simulink library "WaveformsLib"  (Simulink 7.7)
settings: Solver=ode45  SolverMode=SingleTasking  StartTime=0.0  StopTime=10.0  RelTol=1e-3
undefined symbols (not defined in the file or in its folder): etaZ, EX, gainZ, gammaZ, mgZ, tauFall, tauFZ, tauRise, tauRZ, tauX
libraries: SpikingLib x10, WaveformsLib x6, simulink x3
settings Model: Creator=jpalma  LastModifiedBy=jpalma

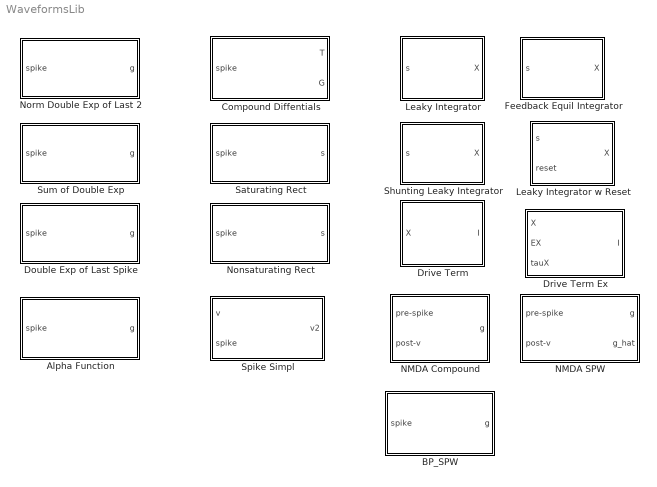
== system WaveformsLib ==
  Alpha Function : Subsystem  mask{tauDecay=2, onsetStr=1}
      mask prompts: tauDecay "Decay Time"; onsetStr "Onset Amplitude"
      mask help: Author: Jesse Palma
      mask Help: Author: Jesse Palma
      mask Display: image(imread('../Libs/icons/AlphaFunct.jpg'),'center');
  BP_SPW : Subsystem  mask{tRise=5, tFall=15, tBP=25, gBP=0.059}
      mask prompts: tRise "Tau Rise Time"; tFall "Tau Fall Time"; tBP "BP Width"; gBP "BP Gain"
      mask help:
      | dT/dt =  - T/tauRise + I * (1-T)
      | dG/dt =  - G/tauFall + T * (1-G)
      |
      | Author: Jesse Palma
      mask Help:
      | dT/dt =  - T/tauRise + I * (1-T)
      | dG/dt =  - G/tauFall + T * (1-G)
      | 
      | Author: Jesse Palma
      mask Display: image(imread('../Libs/icons/DoubleExp.jpg'),'center');
  Compound Diffentials : Subsystem  mask{tauRise=0.78, tauFall=6.5, squareWaveWidth=0.5, squareWaveHeight=2, interGain=1, finalGain=1}
      mask prompts: tauRise "Tau Rise Time"; tauFall "Tau Fall Time"; squareWaveWidth "Square Wave Width"; squareWaveHeight "Square Wave Height"; interGain "Intermediate Gain"; finalGain "Final Gain"
      mask help:
      | dT/dt =  - T/tauRise + I * (1-T)
      | dG/dt =  - G/tauFall + T * (1-G)
      |
      | Author: Jesse Palma
      mask Help:
      | dT/dt =  - T/tauRise + I * (1-T)
      | dG/dt =  - G/tauFall + T * (1-G)
      | 
      | Author: Jesse Palma
      mask Display: image(imread('../Libs/icons/DoubleExp.jpg'),'center');
  Double Exp of Last Spike : Subsystem  mask{tauRise=1, tauFall=2}
      mask prompts: tauRise "Tau Rise Time"; tauFall "Tau Fall Time"
      mask help: Author: Jesse Palma
      mask Help: Author: Jesse Palma
      mask Display: image(imread('../Libs/icons/DoubleExp.jpg'),'center');
  Drive Term : Subsystem  mask{EX=EX, tauX=tauX}
      mask prompts: EX "Equilibrium, EX"; tauX "Rate Time Constant, tauX"
      mask help: IX = 1/tauX (EX - X)
      mask Help: IX =  1/tauX (EX - X)
      mask Display: image(imread('../Libs/icons/DriveArrow.jpg'),'center');
  Drive Term Ex : Subsystem
      mask Description: IX =  1/tauX (EX - X)
      mask Help: IX =  1/tauX (EX - X)
      mask Display: image(imread('../Libs/icons/DriveArrow.jpg'),'center');
  Feedback Equil Integrator : Subsystem  mask{X0=0, A=0.05, EX=0}
      mask prompts: X0 "Initial Value, X0"; A "Decay Rate, A"; EX "Equilbrium (Rest) Value, EX"
      mask help:
      | dX/dt =  - A(EX - X) + s
      |
      | Author: Jesse Palma
      mask Help:
      | dX/dt =  - A(EX - X) + s
      | 
      | Author: Jesse Palma
      mask Display: image(imread('../Libs/icons/FeedbackEq.jpg'),'center');
  Leaky Integrator : Subsystem  mask{X0=0, A=0.05}
      mask prompts: X0 "Initial Value, X0"; A "Decay Rate, A"
      mask help: Author: Jesse Palma
      mask Help: Author: Jesse Palma
      mask Display: image(imread('../Libs/icons/Leaky.jpg'),'center');
  Leaky Integrator w Reset : Subsystem  mask{X0=0, A=0.05}
      mask prompts: X0 "Initial Value, X0"; A "Decay Rate, A"
      mask help: Author: Jesse Palma
      mask Help: Author: Jesse Palma
      mask Display: image(imread('../Libs/icons/Leaky.jpg'),'center');
  NMDA Compound : Subsystem  mask{rt=0.5, ft=40, eta=0.33, mg=1, gamma=0.06, gn=4}
      mask prompts: rt "Rise Time"; ft "Fall Time"; eta "Voltage-dependence, eta"; mg "Mg concentration"; gamma "Voltage-chandge-dependence, gamma"; gn "Concentration Gain, gN"
      mask Display: image(imread('../Libs/icons/DoubleExp.jpg'),'center');
  NMDA SPW : Subsystem  mask{tRise=tauRZ, tFall=tauFZ, eta=etaZ, mg=mgZ, gamma=gammaZ, gn=gainZ}
      mask prompts: tRise "Rise Time"; tFall "Fall Time"; eta "Voltage-dependence, eta"; mg "Mg concentration"; gamma "Voltage-chandge-dependence, gamma"; gn "Concentration Gain, gN"
      mask Display: image(imread('../Libs/icons/DoubleExp.jpg'),'center');
  Nonsaturating Rect : Subsystem  AncestorBlock=SpikeToWavesLib/Saturating Rectangular Wave  mask{squareWidth=1, squareHeight=1}
      mask prompts: squareWidth "Rectangular Width"; squareHeight "Rectangular Height"
      mask help: Author: Jesse Palma
      mask Help: Author: Jesse Palma
      mask Display: image(imread('../Libs/icons/SquareWave.jpg'),'center');
  Norm Double Exp of Last 2 : Subsystem  mask{tauRise=tauRise, tauFall=tauFall}
      mask prompts: tauRise "Tau Rise Time"; tauFall "Tau Fall Time"
      mask help:
      | Kinness Style
      |
      | Author: Jesse Palma
      mask Help:
      | Kinness Style
      | 
      | Author: Jesse Palma
      mask Display: image(imread('../Libs/icons/DoubleExp.jpg'),'center');
  Saturating Rect : Subsystem  mask{squareWidth=1, squareHeight=1}
      mask prompts: squareWidth "Rectangular Width"; squareHeight "Rectangular Height"
      mask help: Author: Jesse Palma
      mask Help: Author: Jesse Palma
      mask Display: image(imread('../Libs/icons/SquareWave.jpg'),'center');
  Shunting Leaky Integrator : Subsystem  mask{X0=0, A=0.05, B=1}
      mask prompts: X0 "Initial Value, X0"; A "Decay Rate, A"; B "Saturation Value, B"
      mask help: Author: Jesse Palma
      mask Help: Author: Jesse Palma
      mask Display: image(imread('../Libs/icons/SLeaky.jpg'),'center');
  Spike Simpl : Subsystem  mask{a=-0.2, b=0.65, c=0.002}
      mask prompts: a "A, drop slope"; b "B, max"; c "C, recovery slope"
      mask help: Author: Jesse Palma
      mask Help: Author: Jesse Palma
      mask Display: image(imread('../Libs/icons/SpikeSimp1.jpg'),'center');
  Sum of Double Exp : Subsystem  mask{tauRise=0.78, tauFall=6.5, timeStep=0.01}
      mask prompts: tauRise "Tau Rise Time"; tauFall "Tau Fall Time"; timeStep "Time Step"
      mask help: Author: Jesse Palma
      mask Help: Author: Jesse Palma
      mask Display: image(imread('../Libs/icons/DoubleExp.jpg'),'center');

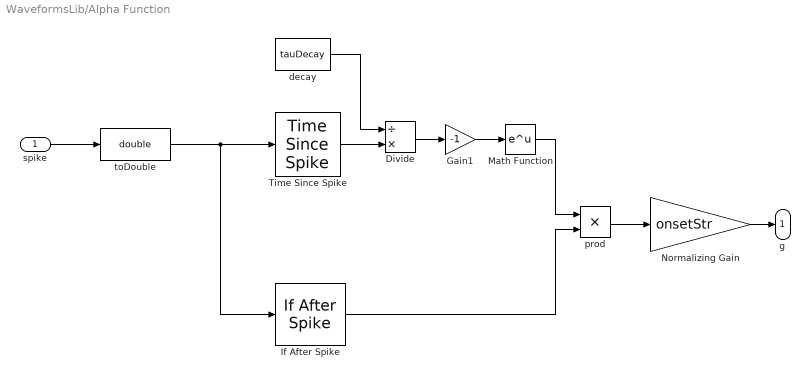
== system WaveformsLib/Alpha Function ==
  spike : Inport
  Divide : Product  Inputs=/*
  Gain1 : Gain  Gain=-1
  If After Spike : SpikingLib/If After Spike  SystemSampleTime=-1
  Math Function : Math  SaturateOnIntegerOverflow=on
  Normalizing Gain : Gain  Gain=onsetStr
  Time Since Spike : SpikingLib/Time Since Spike  SystemSampleTime=-1
  decay : Constant  Value=tauDecay
  prod : Product  Inputs=**
  toDouble : DataTypeConversion  OutDataTypeStr=double
  g : Outport
  wires:
  Normalizing Gain/1 -> g/1
  prod/1 -> Normalizing Gain/1
  spike/1 -> toDouble/1
  toDouble/1 -> Time Since Spike/1, If After Spike/1
  Gain1/1 -> Math Function/1
  Divide/1 -> Gain1/1
  decay/1 -> Divide/1
  Time Since Spike/1 -> Divide/2
  Math Function/1 -> prod/1
  If After Spike/1 -> prod/2

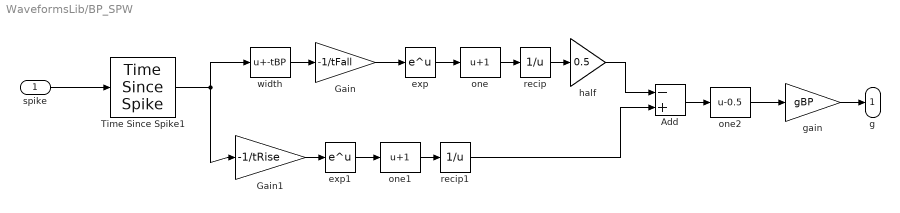
== system WaveformsLib/BP_SPW ==
  spike : Inport
  Add : Sum  Inputs=-+
  Gain : Gain  Gain=-1/tFall
  Gain1 : Gain  Gain=-1/tRise
  Time Since Spike1 : SpikingLib/Time Since Spike  SystemSampleTime=-1
  exp : Math  SaturateOnIntegerOverflow=on
  exp1 : Math  SaturateOnIntegerOverflow=on
  gain : Gain  Gain=gBP
  half : Gain  Gain=0.5
  one : Bias  Bias=1
  one1 : Bias  Bias=1
  one2 : Bias  Bias=-0.5
  recip : Math  Operator=reciprocal  SaturateOnIntegerOverflow=on
  recip1 : Math  Operator=reciprocal  SaturateOnIntegerOverflow=on
  width : Bias  Bias=-tBP
  g : Outport
  wires:
  spike/1 -> Time Since Spike1/1
  width/1 -> Gain/1
  Time Since Spike1/1 -> width/1, Gain1/1
  Gain/1 -> exp/1
  exp/1 -> one/1
  one/1 -> recip/1
  one1/1 -> recip1/1
  exp1/1 -> one1/1
  Gain1/1 -> exp1/1
  recip/1 -> half/1
  recip1/1 -> Add/2
  half/1 -> Add/1
  Add/1 -> one2/1
  one2/1 -> gain/1
  gain/1 -> g/1

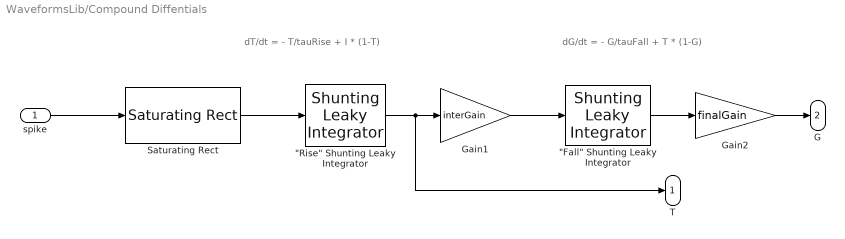
== system WaveformsLib/Compound Diffentials ==
  note: dT/dt = - T/tauRise + I * (1-T)
  note: dG/dt = - G/tauFall + T * (1-G)
  spike : Inport
  "\"Fall\" Shunting Leaky Integrator" : WaveformsLib/Shunting Leaky Integrator  SystemSampleTime=-1  X0=0  A=1/tauFall  B=1
  "\"Rise\" Shunting Leaky Integrator" : WaveformsLib/Shunting Leaky Integrator  SystemSampleTime=-1  X0=0  A=1/tauRise  B=1
  Gain1 : Gain  Gain=interGain
  Gain2 : Gain  Gain=finalGain
  Saturating Rect : WaveformsLib/Saturating Rect  SystemSampleTime=-1  squareWidth=squareWaveWidth  squareHeight=squareWaveHeight
  T : Outport
  G : Outport  Port=2
  wires:
  Gain2/1 -> G/1
  spike/1 -> Saturating Rect/1
  Saturating Rect/1 -> "\"Rise\" Shunting Leaky Integrator"/1
  "\"Rise\" Shunting Leaky Integrator"/1 -> Gain1/1, T/1
  Gain1/1 -> "\"Fall\" Shunting Leaky Integrator"/1
  "\"Fall\" Shunting Leaky Integrator"/1 -> Gain2/1

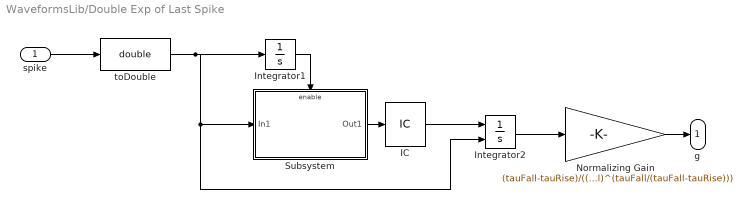
== system WaveformsLib/Double Exp of Last Spike ==
  spike : Inport
  IC : InitialCondition  Value=0
  Integrator1 : Integrator
  Integrator2 : Integrator  ExternalReset=rising
  Normalizing Gain : Gain  Gain=(tauFall-tauRise)/((tauRise/tauFall)^(tauRise/(tauFall-tauRise)) - (tauRise/tauFall)^(tauFall/(tauFall-tauRise)))
  Subsystem : Subsystem
  toDouble : DataTypeConversion  OutDataTypeStr=double
  g : Outport
  wires:
  Integrator1/1 -> Subsystem/Enable
  IC/1 -> Integrator2/1
  toDouble/1 -> Integrator2/2, Subsystem/1(In1), Integrator1/1
  spike/1 -> toDouble/1
  Subsystem/1(Out1) -> IC/1
  Integrator2/1 -> Normalizing Gain/1
  Normalizing Gain/1 -> g/1

== system WaveformsLib/Drive Term ==
  note: I_{X} = 1/tau_{X} (E_{X} - X)
  X : Inport
  XEq1 : Bias  Bias=-EX
  XGain : Gain  Gain=-1/tauX
  I : Outport
  wires:
  XGain/1 -> I/1
  XEq1/1 -> XGain/1
  X/1 -> XEq1/1

== system WaveformsLib/Drive Term Ex ==
  note: I_{X} = 1/tau_{X} (E_{X} - X)
  X : Inport
  EX : Inport  Port=2
  tauX : Inport  Port=3
  Add : Sum  Inputs=-+
  Product : Product  Inputs=*/  RndMeth=Zero
  I : Outport
  wires:
  X/1 -> Add/1
  EX/1 -> Add/2
  Product/1 -> I/1
  Add/1 -> Product/1
  tauX/1 -> Product/2

== system WaveformsLib/Feedback Equil Integrator ==
  note: dX/dt = - A(E_X - X) + s
  s : Inport
  Add : Sum  Inputs=+-
  Drive Term : WaveformsLib/Drive Term  SystemSampleTime=-1  EX=EX  tauX=1/A
  Integrate X : Integrator  InitialCondition=X0
  X : Outport
  wires:
  s/1 -> Add/1
  Integrate X/1 -> X/1, Drive Term/1
  Add/1 -> Integrate X/1
  Drive Term/1 -> Add/2

== system WaveformsLib/Leaky Integrator ==
  note: dX/dt = - AX + s
  note: Decay
  s : Inport
  Add : Sum  Inputs=+-
  Gain1 : Gain  Gain=A
  Integrate X : Integrator  InitialCondition=X0
  X : Outport
  wires:
  Gain1/1 -> Add/2
  Add/1 -> Integrate X/1
  Integrate X/1 -> Gain1/1, X/1
  s/1 -> Add/1

== system WaveformsLib/Leaky Integrator w Reset ==
  note: Decay
  note: dX/dt = - AX + s
  s : Inport
  reset : Inport  Port=2
  Add : Sum  Inputs=+-
  Gain1 : Gain  Gain=A
  Integrate X : Integrator  ExternalReset=falling  InitialCondition=X0
  X : Outport
  wires:
  s/1 -> Add/1
  Integrate X/1 -> X/1, Gain1/1
  Add/1 -> Integrate X/1
  Gain1/1 -> Add/2
  reset/1 -> Integrate X/2

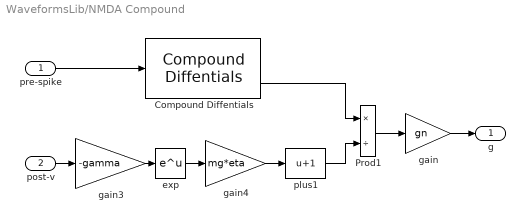
== system WaveformsLib/NMDA Compound ==
  pre-spike : Inport
  post-v : Inport  Port=2
  Compound Diffentials : WaveformsLib/Compound Diffentials  SystemSampleTime=-1  tauRise=rt  tauFall=ft  squareWaveWidth=0.5  squareWaveHeight=2  interGain=1  finalGain=1
  Prod1 : Product  Inputs=*/  RndMeth=Zero
  exp : Math  SaturateOnIntegerOverflow=on
  gain : Gain  Gain=gn
  gain3 : Gain  Gain=-gamma
  gain4 : Gain  Gain=mg*eta
  plus1 : Bias  Bias=1
  g : Outport
  wires:
  Compound Diffentials/2 -> Prod1/1
  gain3/1 -> exp/1
  exp/1 -> gain4/1
  gain4/1 -> plus1/1
  plus1/1 -> Prod1/2
  Prod1/1 -> gain/1
  pre-spike/1 -> Compound Diffentials/1
  post-v/1 -> gain3/1
  gain/1 -> g/1

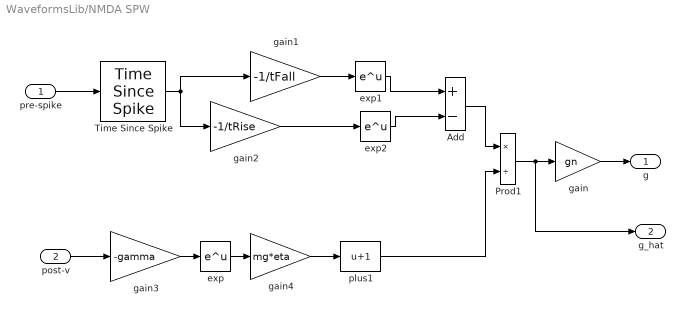
== system WaveformsLib/NMDA SPW ==
  pre-spike : Inport
  post-v : Inport  Port=2
  Add : Sum  Inputs=+-
  Prod1 : Product  Inputs=*/  RndMeth=Zero
  Time Since Spike : SpikingLib/Time Since Spike  SystemSampleTime=-1
  exp : Math  SaturateOnIntegerOverflow=on
  exp1 : Math  SaturateOnIntegerOverflow=on
  exp2 : Math  SaturateOnIntegerOverflow=on
  gain : Gain  Gain=gn
  gain1 : Gain  Gain=-1/tFall
  gain2 : Gain  Gain=-1/tRise
  gain3 : Gain  Gain=-gamma
  gain4 : Gain  Gain=mg*eta
  plus1 : Bias  Bias=1
  g : Outport
  g_hat : Outport  Port=2
  wires:
  gain/1 -> g/1
  post-v/1 -> gain3/1
  pre-spike/1 -> Time Since Spike/1
  Prod1/1 -> gain/1, g_hat/1
  plus1/1 -> Prod1/2
  gain4/1 -> plus1/1
  exp/1 -> gain4/1
  gain3/1 -> exp/1
  Add/1 -> Prod1/1
  gain1/1 -> exp1/1
  gain2/1 -> exp2/1
  exp1/1 -> Add/1
  exp2/1 -> Add/2
  Time Since Spike/1 -> gain1/1, gain2/1

== system WaveformsLib/Nonsaturating Rect ==
  spike : Inport
  Gain : Gain  Gain=squareHeight
  SpikeCounter : SpikingLib/SpikeCounter  SystemSampleTime=-1
  Subtract : Sum  Inputs=+-
  Transport Delay : TransportDelay  DelayTime=squareWidth
  s : Outport
  wires:
  Gain/1 -> s/1
  spike/1 -> SpikeCounter/1
  SpikeCounter/1 -> Subtract/1, Transport Delay/1
  Transport Delay/1 -> Subtract/2
  Subtract/1 -> Gain/1

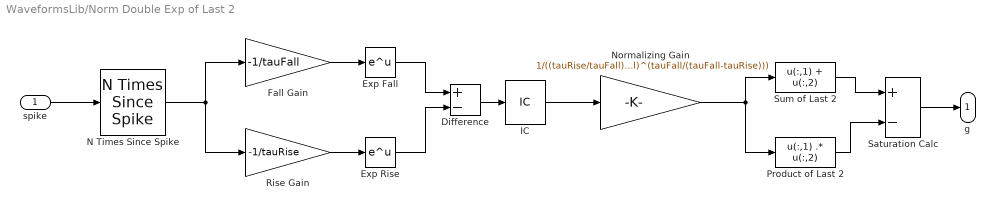
== system WaveformsLib/Norm Double Exp of Last 2 ==
  spike : Inport
  Difference : Sum  Inputs=+-
  Exp Fall : Math  SaturateOnIntegerOverflow=on
  Exp Rise : Math  SaturateOnIntegerOverflow=on
  Fall Gain : Gain  Gain=-1/tauFall
  IC : InitialCondition  Value=0
  N Times Since Spike : SpikingLib/N Times Since Spike  SystemSampleTime=-1  spikesMemory=2
  Normalizing Gain : Gain  Gain=1/((tauRise/tauFall)^(tauRise/(tauFall-tauRise)) - (tauRise/tauFall)^(tauFall/(tauFall-tauRise)))
  Product of Last 2 : MATLABFcn  MATLABFcn="u(:,1) .*  u(:,2)"
  Rise Gain : Gain  Gain=-1/tauRise
  Saturation Calc : Sum  Inputs=+-
  Sum of Last 2 : MATLABFcn  MATLABFcn=u(:,1) + u(:,2)
  g : Outport
  wires:
  Product of Last 2/1 -> Saturation Calc/2
  Sum of Last 2/1 -> Saturation Calc/1
  Normalizing Gain/1 -> Product of Last 2/1, Sum of Last 2/1
  Exp Rise/1 -> Difference/2
  Exp Fall/1 -> Difference/1
  Fall Gain/1 -> Exp Fall/1
  Rise Gain/1 -> Exp Rise/1
  Saturation Calc/1 -> g/1
  spike/1 -> N Times Since Spike/1
  IC/1 -> Normalizing Gain/1
  Difference/1 -> IC/1
  N Times Since Spike/1 -> Rise Gain/1, Fall Gain/1

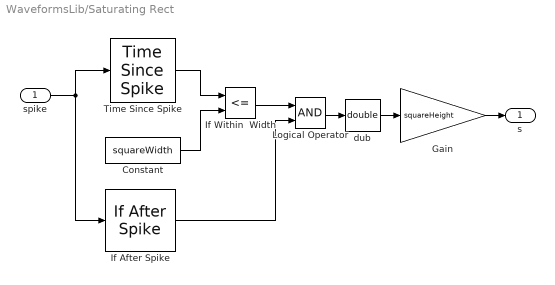
== system WaveformsLib/Saturating Rect ==
  spike : Inport
  Constant : Constant  Value=squareWidth
  Gain : Gain  Gain=squareHeight
  If After Spike : SpikingLib/If After Spike  SystemSampleTime=-1
  If Within  Width : RelationalOperator  Operator=<=  OutDataTypeStr=boolean
  Logical Operator : Logic  AllPortsSameDT=off  OutDataTypeStr=boolean
  Time Since Spike : SpikingLib/Time Since Spike  SystemSampleTime=-1
  dub : DataTypeConversion  OutDataTypeStr=double
  s : Outport
  wires:
  Logical Operator/1 -> dub/1
  Constant/1 -> If Within  Width/2
  If After Spike/1 -> Logical Operator/2
  If Within  Width/1 -> Logical Operator/1
  Time Since Spike/1 -> If Within  Width/1
  spike/1 -> Time Since Spike/1, If After Spike/1
  Gain/1 -> s/1
  dub/1 -> Gain/1

== system WaveformsLib/Shunting Leaky Integrator ==
  note: dX/dt = - AX + s * (B-X)
  s : Inport
  Leaky Integrator : WaveformsLib/Leaky Integrator  SystemSampleTime=-1  X0=X0  A=A
  Max Bias : Bias  Bias=B
  Product : Product  RndMeth=Zero
  Unary Minus : UnaryMinus
  X : Outport
  wires:
  s/1 -> Product/1
  Leaky Integrator/1 -> X/1, Unary Minus/1
  Product/1 -> Leaky Integrator/1
  Unary Minus/1 -> Max Bias/1
  Max Bias/1 -> Product/2

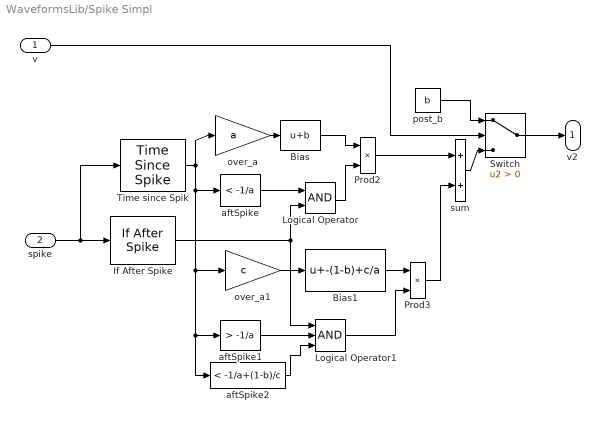
== system WaveformsLib/Spike Simpl ==
  v : Inport
  spike : Inport  Port=2
  Bias : Bias  Bias=b
  Bias1 : Bias  Bias=-(1-b)+c/a
  If After Spike : SpikingLib/If After Spike  SystemSampleTime=-1
  Logical Operator : Logic  AllPortsSameDT=off  OutDataTypeStr=boolean
  Logical Operator1 : Logic  Inputs=3  AllPortsSameDT=off  OutDataTypeStr=boolean
  Prod2 : Product  RndMeth=Zero
  Prod3 : Product  RndMeth=Zero
  Switch : Switch  Criteria=u2 > Threshold  ZeroCross=off
  Time since Spik : SpikingLib/Time Since Spike  SystemSampleTime=-1
  aftSpike : simulink/Logic and Bit Operations/Compare To Constant  SystemSampleTime=-1  relop=<  const=-1/a  LogicOutDataTypeMode=uint8  ZeroCross=off
  aftSpike1 : simulink/Logic and Bit Operations/Compare To Constant  SystemSampleTime=-1  relop=>  const=-1/a  LogicOutDataTypeMode=uint8  ZeroCross=off
  aftSpike2 : simulink/Logic and Bit Operations/Compare To Constant  SystemSampleTime=-1  relop=<  const=-1/a+(1-b)/c  LogicOutDataTypeMode=uint8  ZeroCross=off
  over_a : Gain  Gain=a
  over_a1 : Gain  Gain=c
  post_b : Constant  Value=b
  sum : Sum
  v2 : Outport
  wires:
  Switch/1 -> v2/1
  v/1 -> Switch/2
  Time since Spik/1 -> over_a/1, aftSpike/1, over_a1/1, aftSpike1/1, aftSpike2/1
  over_a/1 -> Bias/1
  Bias/1 -> Prod2/1
  aftSpike/1 -> Logical Operator/1
  If After Spike/1 -> Logical Operator/2, Logical Operator1/1
  Logical Operator/1 -> Prod2/2
  over_a1/1 -> Bias1/1
  aftSpike2/1 -> Logical Operator1/3
  aftSpike1/1 -> Logical Operator1/2
  Bias1/1 -> Prod3/1
  Logical Operator1/1 -> Prod3/2
  Prod3/1 -> sum/2
  Prod2/1 -> sum/1
  sum/1 -> Switch/3
  post_b/1 -> Switch/1
  spike/1 -> Time since Spik/1, If After Spike/1

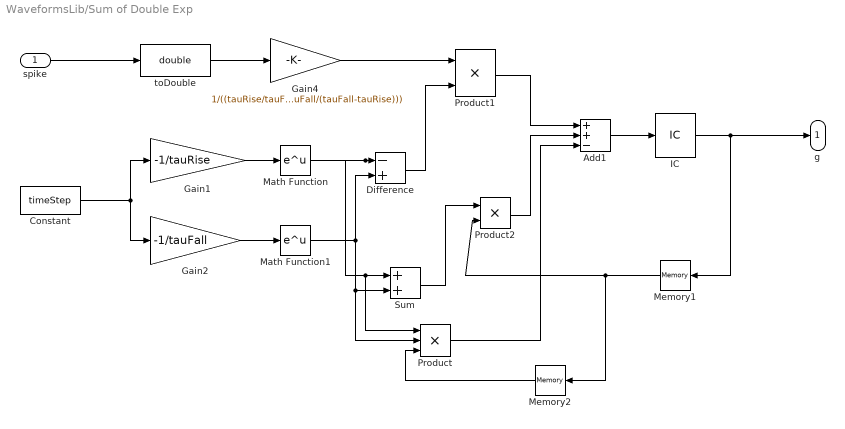
== system WaveformsLib/Sum of Double Exp ==
  spike : Inport
  Add1 : Sum  Inputs=++-
  Constant : Constant  Value=timeStep
  Difference : Sum  Inputs=-+
  Gain1 : Gain  Gain=-1/tauRise
  Gain2 : Gain  Gain=-1/tauFall
  Gain4 : Gain  Gain=1/((tauRise/tauFall)^(tauRise/(tauFall-tauRise)) - (tauRise/tauFall)^(tauFall/(tauFall-tauRise)))
  IC : InitialCondition  Value=0
  Math Function : Math  SaturateOnIntegerOverflow=on
  Math Function1 : Math  SaturateOnIntegerOverflow=on
  Memory1 : Memory
  Memory2 : Memory
  Product : Product  Inputs=3  RndMeth=Zero
  Product1 : Product  Inputs=**  RndMeth=Zero
  Product2 : Product  RndMeth=Zero
  Sum : Sum
  toDouble : DataTypeConversion  OutDataTypeStr=double
  g : Outport
  wires:
  Difference/1 -> Product1/2
  Product2/1 -> Add1/2
  Product/1 -> Add1/3
  Memory2/1 -> Product/3
  Sum/1 -> Product2/1
  Memory1/1 -> Product2/2, Memory2/1
  IC/1 -> g/1, Memory1/1
  Add1/1 -> IC/1
  Product1/1 -> Add1/1
  Math Function1/1 -> Product/2, Sum/2, Difference/2
  Math Function/1 -> Product/1, Sum/1, Difference/1
  Gain2/1 -> Math Function1/1
  Gain1/1 -> Math Function/1
  toDouble/1 -> Gain4/1
  spike/1 -> toDouble/1
  Gain4/1 -> Product1/1
  Constant/1 -> Gain1/1, Gain2/1

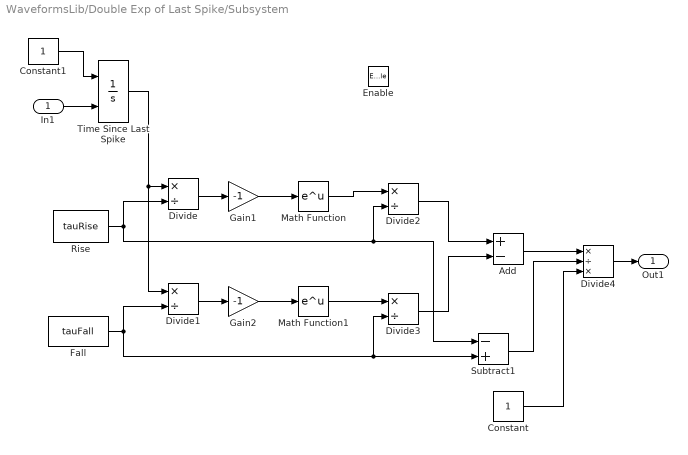
== system WaveformsLib/Double Exp of Last Spike/Subsystem ==
  In1 : Inport
  Enable : EnablePort
  Add : Sum  Inputs=+-
  Constant : Constant
  Constant1 : Constant
  Divide{,1..3} (4 alike) : Product  Inputs=*/
  Divide4 : Product  Inputs=*/*
  Fall : Constant  Value=tauFall
  Gain1 : Gain  Gain=-1
  Gain2 : Gain  Gain=-1
  Math Function : Math  SaturateOnIntegerOverflow=on
  Math Function1 : Math  SaturateOnIntegerOverflow=on
  Rise : Constant  Value=tauRise
  Subtract1 : Sum  Inputs=-+
  Time Since Last Spike : Integrator  ExternalReset=falling
  Out1 : Outport
  wires:
  Divide4/1 -> Out1/1
  In1/1 -> Time Since Last Spike/2
  Constant/1 -> Divide4/3
  Subtract1/1 -> Divide4/2
  Divide3/1 -> Add/2
  Divide2/1 -> Add/1
  Time Since Last Spike/1 -> Divide1/1, Divide/1
  Add/1 -> Divide4/1
  Math Function1/1 -> Divide3/1
  Math Function/1 -> Divide2/1
  Gain1/1 -> Math Function/1
  Gain2/1 -> Math Function1/1
  Divide/1 -> Gain1/1
  Divide1/1 -> Gain2/1
  Fall/1 -> Divide1/2, Divide3/2, Subtract1/2
  Rise/1 -> Divide/2, Divide2/2, Subtract1/1
  Constant1/1 -> Time Since Last Spike/1
